simulink model "test"  (Simulink 7.4)
settings: Solver=ode45  StartTime=0.0  StopTime=10.0  RelTol=1e-3
values from neighbouring files (symbols this model uses):
  x_init_lin = [0.898 ... (first row only)    [MpcSetup.m]    (also in MpcSetup_linearized.m; compressor_setup.m; setup_compressor.m; test2.m = [0.899; 1.125; 0.1512; 440.7; 0])
settings Model: Creator=CHKAJON  LastModifiedBy=CHKAJON

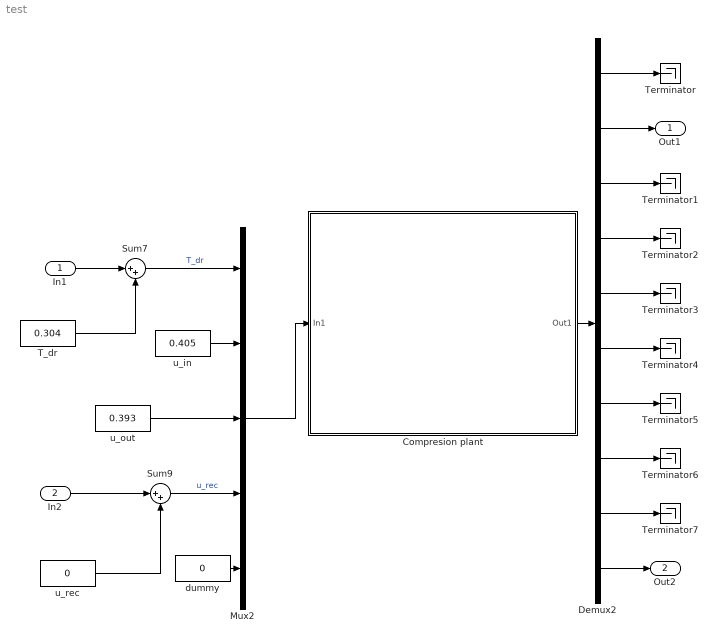
== system test ==
  In1 : Inport
  In2 : Inport  Port=2
  Compresion plant : Subsystem
      mask Display: image(imread('comp_plant.jpg'))
  Demux2 : Demux  Outputs=10
  Mux2 : Mux  Inputs=5
  Sum7 : Sum  Inputs=|++
  Sum9 : Sum  Inputs=|++
  T_dr : Constant  Value=0.304
  Terminator{,1..7} (8 alike) : Terminator
  dummy : Constant  Value=0
  u_in : Constant  Value=0.405
  u_out : Constant  Value=0.393
  u_rec : Constant  Value=0
  Out1 : Outport
  Out2 : Outport  Port=2
  wires:
  dummy/1 -> Mux2/5
  In1/1 -> Sum7/1
  u_rec/1 -> Sum9/2
  T_dr/1 -> Sum7/2
  Sum9/1 -> Mux2/4  "u_rec"
  Sum7/1 -> Mux2/1  "T_dr"
  In2/1 -> Sum9/1
  u_out/1 -> Mux2/3
  u_in/1 -> Mux2/2
  Mux2/1 -> Compresion plant/1(In1)
  Demux2/1 -> Terminator/1
  Demux2/2 -> Out1/1
  Demux2/3 -> Terminator1/1
  Demux2/4 -> Terminator2/1
  Demux2/5 -> Terminator3/1
  Demux2/6 -> Terminator4/1
  Demux2/7 -> Terminator5/1
  Demux2/8 -> Terminator6/1
  Demux2/9 -> Terminator7/1
  Demux2/10 -> Out2/1
  Compresion plant/1(Out1) -> Demux2/1

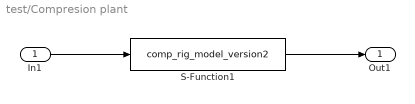
== system test/Compresion plant ==
  In1 : Inport
  S-Function1 : S-Function  FunctionName=comp_rig_model_version2  Parameters=[], x_init_lin  EnableBusSupport=off
  Out1 : Outport
  wires:
  In1/1 -> S-Function1/1
  S-Function1/1 -> Out1/1
